simulink model "demoOtterUSVPathFollowingHeadingControl_own"  (R2020b)
settings: Solver=ode4  StartTime=0.0  StopTime=2000  FixedStep=0.05  RelTol=1e-3
libraries: mssSimulink x5, simulink x1
settings Model: Creator=thor  LastModifiedBy=rapha
settings DebuggingCC: SFMachineParentedDataDiag=error  ArithmeticOperatorsInVariantConditions=warning
settings SFSimCC: CustomCodeUndefinedFunction=UseInterfaceOnly

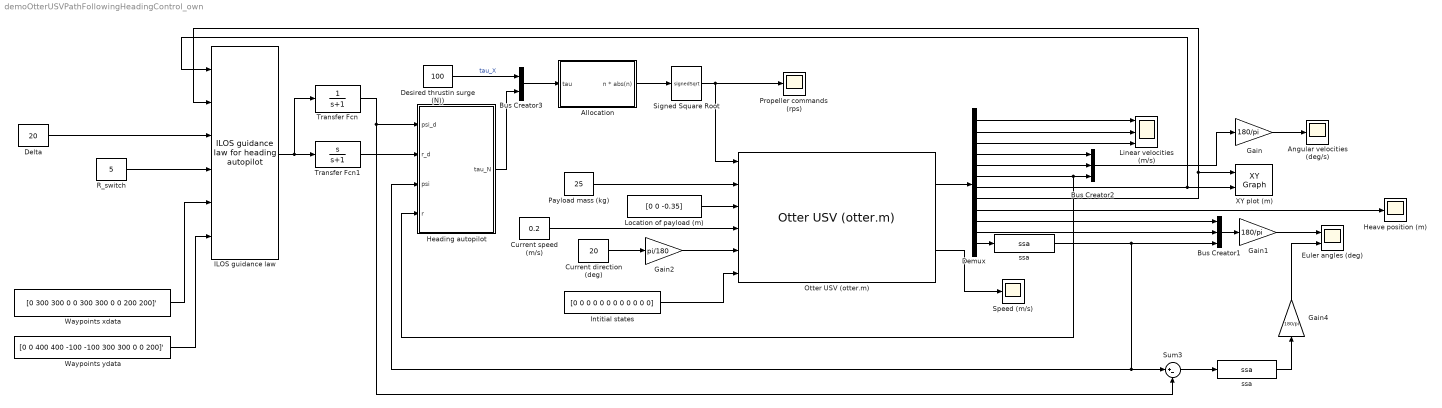
== system demoOtterUSVPathFollowingHeadingControl_own ==
  Allocation : Subsystem
  Angular velocities (deg/s) : Scope
  Bus Creator1 : BusCreator  Inputs=3
  Bus Creator2 : BusCreator  Inputs=3
  Bus Creator3 : BusCreator  Inputs=2
  Current direction (deg) : Constant  Value=20
  Current speed (m/s) : Constant  Value=0.2
  Delta : Constant  Value=20
  Demux : Demux  Outputs=12
  Desired thrustin surge (N)) : Constant  Value=100
  Euler angles (deg) : Scope  NumInputPorts=2
  Gain : Gain  Gain=180/pi
  Gain1 : Gain  Gain=180/pi
  Gain2 : Gain  Gain=pi/180
  Gain4 : Gain  Gain=180/pi
  Heading autopilot : Subsystem
  Heave position (m) : Scope
  ILOS guidance law : mssSimulink/Guidance/ILOS guidance law for heading autopilot  SystemSampleTime=-1  VariantActivationTime=update diagram  Latency=0  AutoFrameSizeCalculation=off
  Intitial states : Constant  Value=[0 0 0 0 0 0 0 0 0 0 0 0]
  Linear velocities (m/s) : Scope  NumInputPorts=3
  Location of payload (m) : Constant  Value=[0 0 -0.35]
  "Otter USV (otter.m) " : mssSimulink/Marine craft models/Otter USV (otter.m)  SystemSampleTime=-1  VariantActivationTime=update diagram  Latency=0  AutoFrameSizeCalculation=off
  Payload mass (kg) : Constant  Value=25
  Propeller commands (rps) : Scope
  R_switch : Constant  Value=5
  Signed Square Root : Sqrt  Operator=signedSqrt  SaturateOnIntegerOverflow=on
  Speed (m/s) : Scope
  Sum3 : Sum  Inputs=|+-  InputSameDT=on  SaturateOnIntegerOverflow=on  OutDataTypeStr=Inherit: Same as first input
  Transfer Fcn : TransferFcn  Denominator=[1 1]
  Transfer Fcn1 : TransferFcn  Numerator=[1 0]  Denominator=[1 1]
  Waypoints xdata : Constant  Value=[0 300 300 0 0 300 300 0 0 200 200]'
  Waypoints ydata : Constant  Value=[0 0 400 400 -100 -100 300 300 0 0 200]'
  XY plot (m) : simulink/Sinks/XY Graph  xmin=-100  xmax=100  ymin=-100  ymax=100  st=-1
  "ssa " : mssSimulink/Utilities/Math Operations/ssa  SystemSampleTime=-1  VariantActivationTime=update diagram  Latency=0  AutoFrameSizeCalculation=off
  "ssa   " : mssSimulink/Utilities/Math Operations/ssa  SystemSampleTime=-1  VariantActivationTime=update diagram  Latency=0  AutoFrameSizeCalculation=off
  wires:
  Demux/1 -> Linear velocities (m/s)/1
  Demux/2 -> Linear velocities (m/s)/2
  Demux/3 -> Linear velocities (m/s)/3
  Demux/10 -> Bus Creator1/1
  Demux/11 -> Bus Creator1/2
  Demux/4 -> Bus Creator2/1
  Demux/5 -> Bus Creator2/2
  Bus Creator2/1 -> Gain/1
  Demux/9 -> Heave position (m)/1
  Payload mass (kg)/1 -> "Otter USV (otter.m) "/2
  Location of payload (m)/1 -> "Otter USV (otter.m) "/3
  Current speed (m/s)/1 -> "Otter USV (otter.m) "/4
  Current direction (deg)/1 -> Gain2/1
  Intitial states/1 -> "Otter USV (otter.m) "/6
  "Otter USV (otter.m) "/1 -> Demux/1
  "Otter USV (otter.m) "/2 -> Speed (m/s)/1
  Gain/1 -> Angular velocities (deg/s)/1
  Gain1/1 -> Euler angles (deg)/1
  Gain2/1 -> "Otter USV (otter.m) "/5
  Heading autopilot/1(tau_N) -> Bus Creator3/2
  Demux/12 -> "ssa   "/1
  Demux/6 -> Bus Creator2/3, Heading autopilot/4(r)
  Desired thrustin surge (N))/1 -> Bus Creator3/1  "tau_X"
  Bus Creator3/1 -> Allocation/1(tau)
  Bus Creator1/1 -> Gain1/1
  R_switch/1 -> ILOS guidance law/4
  Delta/1 -> ILOS guidance law/3
  Demux/7 -> ILOS guidance law/1, XY plot (m)/2
  Demux/8 -> ILOS guidance law/2, XY plot (m)/1
  Waypoints xdata/1 -> ILOS guidance law/5
  Waypoints ydata/1 -> ILOS guidance law/6
  "ssa   "/1 -> Bus Creator1/3, Sum3/1, Heading autopilot/3(psi)
  Allocation/1(n * abs(n)) -> Signed Square Root/1
  Sum3/1 -> "ssa "/1
  "ssa "/1 -> Gain4/1
  Gain4/1 -> Euler angles (deg)/2
  ILOS guidance law/1 -> Transfer Fcn/1, Transfer Fcn1/1
  Signed Square Root/1 -> "Otter USV (otter.m) "/1, Propeller commands (rps)/1
  Transfer Fcn/1 -> Sum3/2, Heading autopilot/1(psi_d)
  Transfer Fcn1/1 -> Heading autopilot/2(r_d)

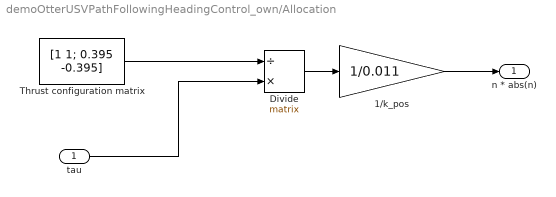
== system demoOtterUSVPathFollowingHeadingControl_own/Allocation ==
  tau : Inport
  1/k_pos : Gain  Gain=1/0.011
  Divide : Product  Inputs=/*  Multiplication=Matrix(*)
  Thrust configuration matrix : Constant  Value=[1 1; 0.395 -0.395]
  n * abs(n) : Outport
  wires:
  1/k_pos/1 -> n * abs(n)/1
  tau/1 -> Divide/2
  Divide/1 -> 1/k_pos/1
  Thrust configuration matrix/1 -> Divide/1

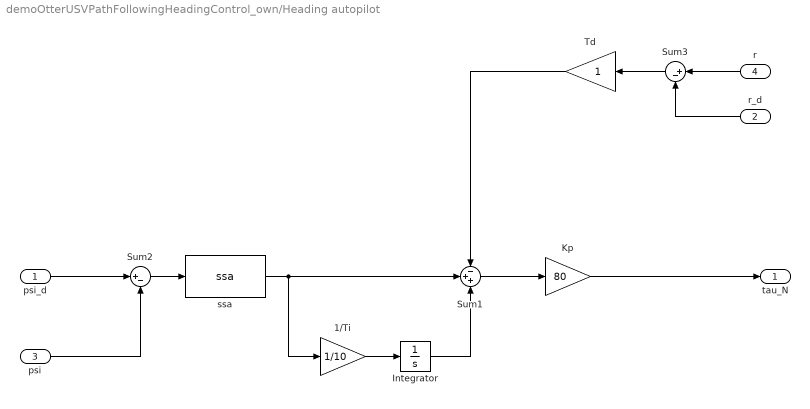
== system demoOtterUSVPathFollowingHeadingControl_own/Heading autopilot ==
  psi_d : Inport
  r_d : Inport  Port=2
  psi : Inport  Port=3
  r : Inport  Port=4
  1/Ti : Gain  Gain=1/10  SaturateOnIntegerOverflow=on  OutDataTypeStr=Inherit: Same as input  ParamDataTypeStr=Inherit: Same as input
  Integrator : Integrator
  Kp : Gain  Gain=80  SaturateOnIntegerOverflow=on  OutDataTypeStr=Inherit: Same as input  ParamDataTypeStr=Inherit: Same as input
  Sum1 : Sum  Inputs=-++  InputSameDT=on  SaturateOnIntegerOverflow=on  OutDataTypeStr=Inherit: Same as first input
  Sum2 : Sum  Inputs=|+-  InputSameDT=on  SaturateOnIntegerOverflow=on  OutDataTypeStr=Inherit: Same as first input
  Sum3 : Sum  Inputs=|+-  InputSameDT=on  SaturateOnIntegerOverflow=on  OutDataTypeStr=Inherit: Same as first input
  Td : Gain  SaturateOnIntegerOverflow=on  OutDataTypeStr=Inherit: Same as input  ParamDataTypeStr=Inherit: Same as input
  "ssa " : mssSimulink/Utilities/Math Operations/ssa  SystemSampleTime=-1  VariantActivationTime=update diagram  Latency=0  AutoFrameSizeCalculation=off
  tau_N : Outport
  wires:
  Td/1 -> Sum1/1
  r/1 -> Sum3/1
  psi/1 -> Sum2/2
  psi_d/1 -> Sum2/1
  Sum2/1 -> "ssa "/1
  Sum1/1 -> Kp/1
  "ssa "/1 -> 1/Ti/1, Sum1/2
  1/Ti/1 -> Integrator/1
  Integrator/1 -> Sum1/3
  Sum3/1 -> Td/1
  Kp/1 -> tau_N/1
  r_d/1 -> Sum3/2
